simulink model "LVDT"  (Simulink 8.0)
settings: Solver=ode4  StartTime=0.0  StopTime=10.0  FixedStep=1e-4  RelTol=1e-3
model workspace (MAT data in the model file):
  lvdt_error = 0
  band = 0
  hyst = 0
  range1 = -1
  range2 = 0
  range3 : num (value not decoded)
settings Model: Creator=HBALLEST  LastModifiedBy=HBALLEST
settings OptimizationCC: InlineParams=on

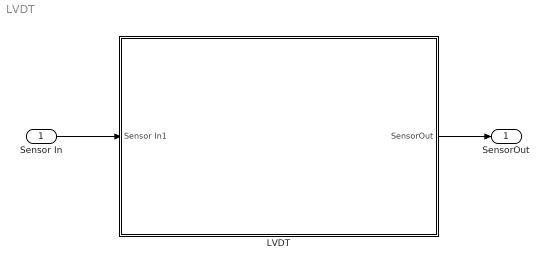
== system LVDT ==
  Sensor In : Inport
  LVDT : Subsystem
  SensorOut : Outport
  wires:
  Sensor In/1 -> LVDT/1(Sensor In1)
  LVDT/1(SensorOut) -> SensorOut/1

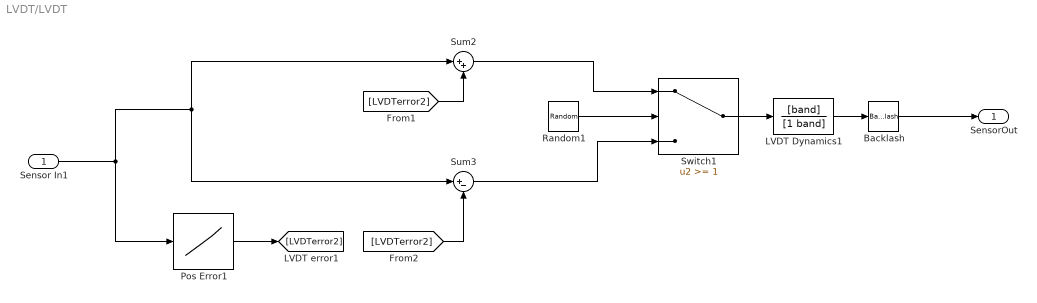
== system LVDT/LVDT ==
  Sensor In1 : Inport
  " Pos Error1" : Lookup_n-D  NumberOfTableDimensions=1  BreakpointsForDimension1=[range1 range2 range3]  Table=[lvdt_error lvdt_error*0.4 lvdt_error]  RndMeth=Simplest  InputSameDT=on
  Backlash : Backlash  BacklashWidth=(range3-range3)*hyst/100
  LVDT Dynamics1 : TransferFcn  Numerator=[band]  Denominator=[1 band]
  Random1 : RandomNumber  Mean=1  Variance=10  SampleTime=1e-4
  Sum2 : Sum  Inputs=|++
  Sum3 : Sum  Inputs=|+-
  Switch1 : Switch  Threshold=1
  SensorOut : Outport
  wires:
  " Pos Error1"/1 -> [LVDTerror2]
  Sum2/1 -> Switch1/1
  Sum3/1 -> Switch1/3
  Backlash/1 -> SensorOut/1
  [LVDTerror2] -> Sum2/2
  Sensor In1/1 -> Sum2/1, Sum3/1, " Pos Error1"/1
  Random1/1 -> Switch1/2
  [LVDTerror2] -> Sum3/2
  LVDT Dynamics1/1 -> Backlash/1
  Switch1/1 -> LVDT Dynamics1/1
